simulink model "PSFBConverter_Simulink"  (R2023b)
settings: Solver=VariableStepAuto  StartTime=0.0  StopTime=0.1  RelTol=1e-3
model workspace (MAT data in the model file):
  PhaseDelay = 0.0005
libraries: spsDiodeLib x4, spsMosfetLib x4, spsSeriesRLCBranchLib x3, spsVoltageMeasurementLib x3, spsDCVoltageSourceLib x1, spsLinearTransformerLib x1, sps_lib x1
settings Model: Creator=Naveen  LastModifiedBy=Naveen

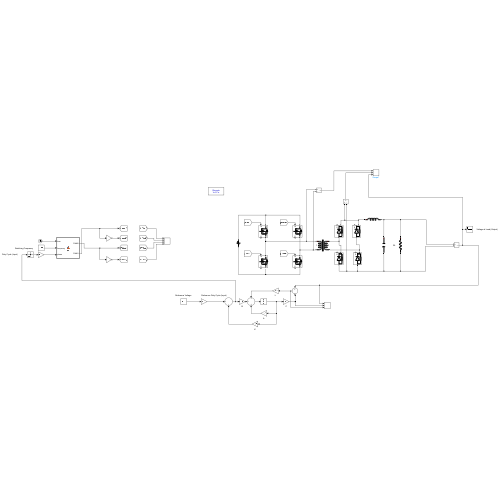
[thumbnail: Simulink's stored preview of the top-level diagram]
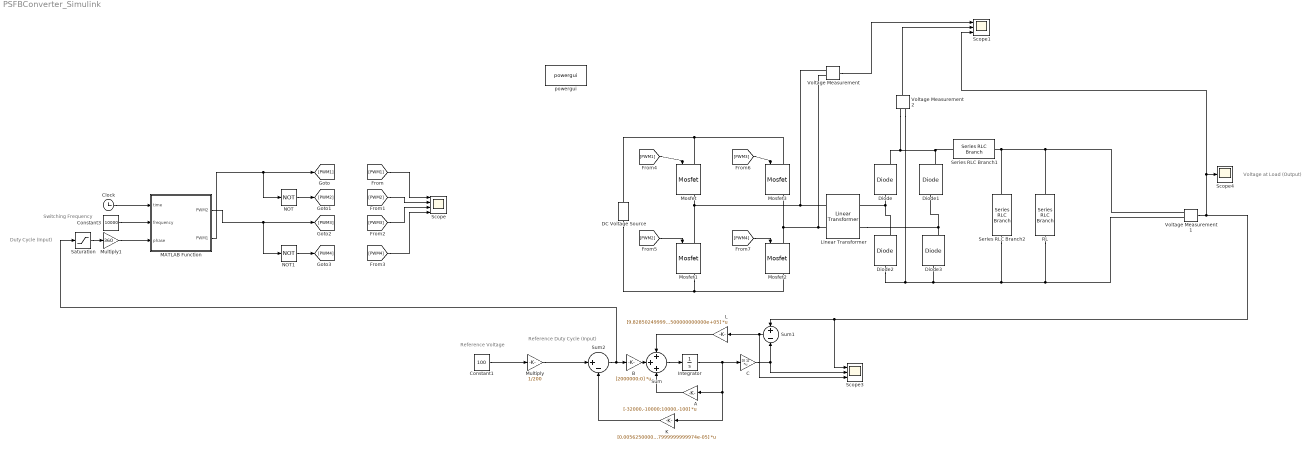
== system PSFBConverter_Simulink ==
  note: Voltage at Load (Output)
  note: Reference Duty Cycle (Input)
  note: Reference Voltage
  note: Duty Cycle (Input)
  note: Switching Frequency
  A : Gain  Gain=[-32000,-10000;10000,-100]  Multiplication=Matrix(K*u)
  B : Gain  Gain=[2000000;0]  Multiplication=Matrix(K*u)
  C : Gain  Gain=[0 1]  Multiplication=Matrix(K*u)
  Clock : Clock
  Constant1 : Constant  Value=100
  Constant3 : Constant  Value=10000
  DC Voltage Source : spsDCVoltageSourceLib/DC Voltage Source  Amplitude=400  Measurements=None
  Diode{,1..3} (4 alike) : spsDiodeLib/Diode  Ron=0.001  Lon=0  Vf=0.8  IC=0  UseSnubber=0  Rs=500  Cs=250e-9  Measurements=on
  Integrator : Integrator
  K : Gain  Gain=[0.005625000000000,-7.877999999999974e-05]  Multiplication=Matrix(K*u)
  L : Gain  Gain=[9.828502499999993e+05;1.156500000000000e+05]  Multiplication=Matrix(K*u)
  Linear Transformer : spsLinearTransformerLib/Linear Transformer  UNITS=SI  NominalPower=[ 2000 50e3 ]  winding1=[400 1e-9 1e-9]  winding2=[100 1e-9 1e-9]  ThreeWindings=off  winding3=[3.15e+05 99225 12.634]  RmLm=[1e6 1e6]  Measurements=None  DataType=on
  MATLAB Function : MATLAB Function  TreatAsAtomicUnit=on
  Mosfet{,1..3} (4 alike) : spsMosfetLib/Mosfet  Ron=0.1  Lon=0  Rd=0.01  Vfd=0  IC=0  Rs=1e5  Cs=inf  Measurements=on
  Multiply : Gain  Gain=1/200
  Multiply1 : Gain  Gain=360
  NOT : Logic  Operator=NOT  IconShape=distinctive  AllPortsSameDT=off  OutDataTypeStr=boolean
  NOT1 : Logic  Operator=NOT  IconShape=distinctive  AllPortsSameDT=off  OutDataTypeStr=boolean
  RL : spsSeriesRLCBranchLib/Series RLC Branch  LConnTagsString=__new0  RConnTagsString=__new0  BranchType=R  Resistance=10  Inductance=1e-3  SetiL0=off  InitialCurrent=0  Capacitance=1e-6  Setx0=off  InitialVoltage=0  Measurements=None
  Saturation : Saturate  LowerLimit=0
  Scope : Scope  NumInputPorts=4
  Scope1 : Scope  NumInputPorts=3
  Scope3 : Scope  NumInputPorts=3
  Scope4 : Scope
  Series RLC Branch1 : spsSeriesRLCBranchLib/Series RLC Branch  LConnTagsString=__new0  RConnTagsString=__new0  BranchType=L  Resistance=0  Inductance=100e-6  SetiL0=off  InitialCurrent=0  Capacitance=0  Setx0=off  InitialVoltage=0  Measurements=None
  Series RLC Branch2 : spsSeriesRLCBranchLib/Series RLC Branch  LConnTagsString=__new0  RConnTagsString=__new0  BranchType=C  Resistance=0  Inductance=5e-6  SetiL0=off  InitialCurrent=0  Capacitance=100e-6  Setx0=off  InitialVoltage=0  Measurements=None
  Sum : Sum  Inputs=+++
  Sum1 : Sum  Inputs=+-
  Sum2 : Sum  Inputs=|+-
  Voltage Measurement : spsVoltageMeasurementLib/Voltage Measurement  PhasorSimulation=off  OutputType=Complex  PSBequivalent=0
  Voltage Measurement1 : spsVoltageMeasurementLib/Voltage Measurement  PhasorSimulation=off  OutputType=Complex  PSBequivalent=0
  Voltage Measurement2 : spsVoltageMeasurementLib/Voltage Measurement  PhasorSimulation=off  OutputType=Complex  PSBequivalent=0
  powergui : sps_lib/powergui  Priority=1  SimulationMode=Discrete  SampleTime=1e-7  frequency=60  Iterations=50  frequencyindice=0  Pbase=100e6  ErrMax=1e-4  UnitsV=kV  UnitsW=MW  buscounter=0  FunctionMessages=off  echomessages=off  EnableUseOfTLC=off  CurrentSourceSwitches=off  DisableSnubberDevices=off  DisableRonSwitches=off  DisableVfSwitches=off  DisplayEquations=off  AutomaticDiscreteSolvers=off  SolverType=Tustin/Backward Euler (TBE)  Interpol=off  ExternalGateDelay=off  methode=off  Ts=100  x0status=blocks  SPID=on  SwTol=0  HookPort=off  NonlinearTolerance=1e-4  nMaxIteration=100  ContinueOnMaxIteration=off  RestoreLinks=warning  ResistiveCurrentMeasurement=off  Frange=[0:2:500]  Ylog=off  Xlog=on  ShowGrid=off  save=off  variable=ZData  structure=0  ZoomFFT=off  StartTime=0.0  cycles=1  DisplayStyle=1  fundamental=60  FreqAxis=off  MaxFrequency=1000  frequencyindicesteady=1  RmsSteady=1  display=off
  wires:
  MATLAB Function/2(PWM1) -> NOT/1, [PWM1]
  NOT/1 -> [PWM2]
  MATLAB Function/1(PWM2) -> NOT1/1, [PWM3]
  NOT1/1 -> [PWM4]
  [PWM1] -> Scope/1
  [PWM2] -> Scope/2
  [PWM3] -> Scope/3
  [PWM4] -> Scope/4
  [PWM1] -> Mosfet/1
  [PWM3] -> Mosfet3/1
  [PWM4] -> Mosfet2/1
  [PWM2] -> Mosfet1/1
  Voltage Measurement/1 -> Scope1/1
  Voltage Measurement1/1 -> Scope1/3, Scope4/1, Scope3/1, Sum1/1
  Voltage Measurement2/1 -> Scope1/2
  B/1 -> Sum/2
  Integrator/1 -> C/1, K/1, A/1
  A/1 -> Sum/3
  Sum/1 -> Integrator/1
  C/1 -> Scope3/2, Sum1/2
  Sum1/1 -> L/1, Scope3/3
  L/1 -> Sum/1
  Clock/1 -> MATLAB Function/1(time)
  Constant3/1 -> MATLAB Function/2(frequency)
  Constant1/1 -> Multiply/1
  Multiply1/1 -> MATLAB Function/3(phase)
  K/1 -> Sum2/2
  Sum2/1 -> Saturation/1, B/1
  Multiply/1 -> Sum2/1
  Saturation/1 -> Multiply1/1
  connections:
  Mosfet1/LConn1 -- Linear Transformer/LConn1 -- Voltage Measurement/LConn1 -- Mosfet/RConn1
  Voltage Measurement/LConn2 -- Linear Transformer/LConn2 -- Mosfet3/RConn1 -- Mosfet2/LConn1
  DC Voltage Source/RConn1 -- Mosfet3/LConn1 -- Mosfet/LConn1
  DC Voltage Source/LConn1 -- Mosfet1/RConn1 -- Mosfet2/RConn1
  Diode2/RConn1 -- Linear Transformer/RConn1 -- Diode/LConn1
  Diode/RConn1 -- Series RLC Branch1/LConn1 -- Diode1/RConn1 -- Voltage Measurement2/LConn1
  Diode2/LConn1 -- RL/RConn1 -- Voltage Measurement1/LConn2 -- Series RLC Branch2/RConn1 -- Diode3/LConn1 -- Voltage Measurement2/LConn2
  Series RLC Branch1/RConn1 -- Voltage Measurement1/LConn1 -- RL/LConn1 -- Series RLC Branch2/LConn1
  Linear Transformer/RConn2 -- Diode1/LConn1 -- Diode3/RConn1

== matlab function PSFBConverter_Simulink/MATLAB Function ==
  data: time input; PWM2 output; frequency input; phase input; PWM1 output
function [PWM2,PWM1] = fcn(time,frequency,phase)
Tswitching = 1/frequency;
PWM1 = 0;
PWM2 = 0;
y1 = mod(time,Tswitching);
if y1<Tswitching/2
    PWM1 = 1;
end

t_phi = Tswitching*phase/360;
y2 = mod(time+t_phi,Tswitching);
if y2<Tswitching/2
    PWM2 = 1;
end
